simulink model "W06_5_offline"  (R2024b)
settings: Solver=ode4  StartTime=0.0  StopTime=80  FixedStep=0.05  RelTol=1e-3
settings Model: Creator=admin  LastModifiedBy=admin

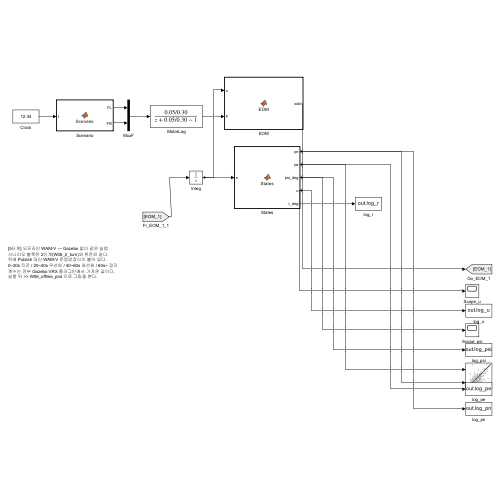
[thumbnail: Simulink's stored preview of the top-level diagram]
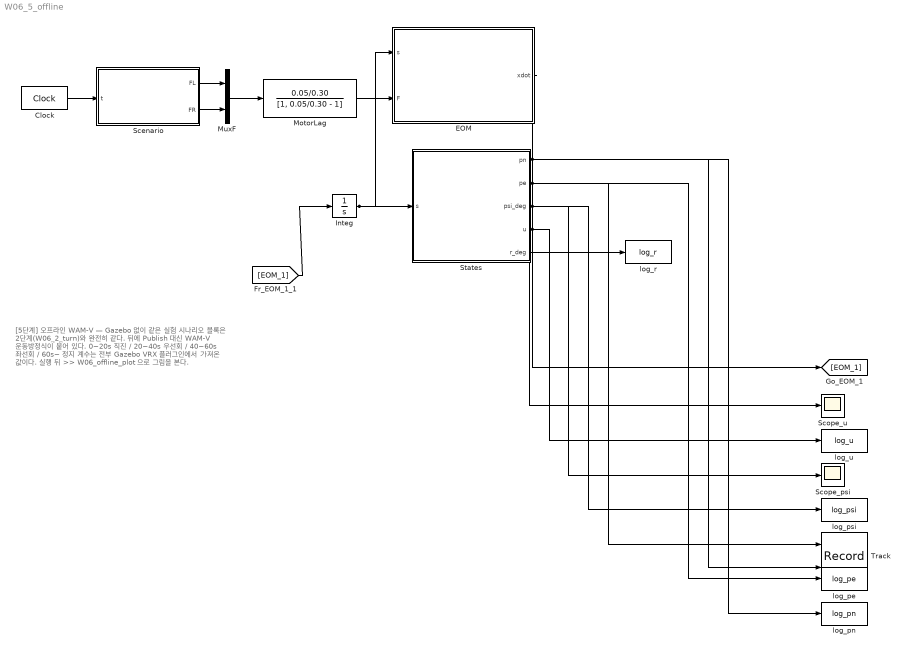
== system W06_5_offline ==
  note: [5단계] 오프라인 WAM-V — Gazebo 없이 같은 실험
      | 시나리오 블록은 2단계(W06_2_turn)와 완전히 같다.
      | 뒤에 Publish 대신 WAM-V 운동방정식이 붙어 있다.
      | 0~20s 직진 / 20~40s 우선회 / 40~60s 좌선회 / 60s~ 정지
      | 계수는 전부 Gazebo VRX 플러그인에서 가져온 값이다.
      | 실행 뒤 >> W06_offline_plot 으로 그림을 본다.
  Clock : DigitalClock  SampleTime=0.05
  EOM : MATLAB Function  TreatAsAtomicUnit=on
  Integ : Integrator  InitialCondition=[0;0;0;0;0;0]
  MotorLag : DiscreteTransferFcn  Numerator=0.05/0.30  Denominator=[1, 0.05/0.30 - 1]  SampleTime=0.05
  MuxF : Mux  Inputs=2
  Scenario : MATLAB Function  TreatAsAtomicUnit=on
  Scope_psi : Scope
  Scope_u : Scope
  States : MATLAB Function  TreatAsAtomicUnit=on
  Track : Record  FileSettingsInternal="{\"entries\":[{\"content\":{\"excelSettings\":{\"content\":{},\"type\":\"Streamout.ExcelSettings\"}},\"type\":\"Streamout.FileSettingStorage\",\"uuid\":\"\"}],\"packageUris\":[\"http:\\/\\/schema.mathworks.com\\/mf0\\/streamout_blocks\\/R2020a\"],\"version\":\"1.0\"}"  Layout=[1 1]  SignalsInternal="{\"entries\":[{\"content\":{\"signals\":[{\"content\":{\"blockPath\":[],\"dimensions\":[1],\"domain\":\"\",\"lineColor\":\"#a2142f\",\"plots\":[ 1 ],\"port\":1,\"signalID\":1,\"signalName\":\"XY Graph:1\"},\"type\":\"RecordBlkView.Signal\",\"uuid\":\"\"},{\"content\":{\"blockPath\":[],\"dimensions\":[1],\"domain\":\"\",\"lineColor\":\"#139fff\",\"plots\":[ 1 ],\"port\":2,\"signalID\":2,\"signalName\":\"XY Graph:2\"},\"type\":\"RecordBlkView.Signal\",\"uuid\":\"\"}]},\"type\":\"RecordBlkView.InputSignals\",\"uuid\":\"\"}],\"packageUris\":[\"http:\\/\\/schema.mathworks.com\\/mf0\\/streamout_blocks\\/R2020a\"],\"version\":\"1.0\"}"  VisualizationBindings="{\"xyplotplugin\":{\"info\":[{\"series\":[{\"bindingParametersList\":[{\"parameter\":\"X-Axis\",\"signalID\":1,\"signalName\":\"XY Graph:1\"},{\"parameter\":\"Y-Axis\",\"signalID\":2,\"signalName\":\"XY Graph:2\"}],\"seriesID\":0}],\"subplotID\":1}]}}"  CompatibilityTag=XY
  log_pe : ToWorkspace  VariableName=log_pe  SaveFormat=Timeseries  SampleTime=0.05
  log_pn : ToWorkspace  VariableName=log_pn  SaveFormat=Timeseries  SampleTime=0.05
  log_psi : ToWorkspace  VariableName=log_psi  SaveFormat=Timeseries  SampleTime=0.05
  log_r : ToWorkspace  VariableName=log_r  SaveFormat=Timeseries  SampleTime=0.05
  log_u : ToWorkspace  VariableName=log_u  SaveFormat=Timeseries  SampleTime=0.05
  wires:
  Clock/1 -> Scenario/1(t)
  Scenario/1(FL) -> MuxF/1
  MotorLag/1 -> EOM/2(F)
  Scenario/2(FR) -> MuxF/2
  MuxF/1 -> MotorLag/1
  Integ/1 -> EOM/1(s), States/1(s)
  States/5(r_deg) -> log_r/1
  [EOM_1] -> Integ/1
  EOM/1(xdot) -> [EOM_1]
  States/4(u) -> Scope_u/1, log_u/1
  States/3(psi_deg) -> Scope_psi/1, log_psi/1
  States/2(pe) -> Track/1, log_pe/1
  States/1(pn) -> Track/2, log_pn/1

== matlab function W06_5_offline/EOM ==
  data: s input; xdot output; F input
function xdot = EOM(s, F)
%#codegen
% 3-DOF WAM-V equations of motion in NED.
% Every coefficient below is taken from the Gazebo VRX plugins, so
% this model and the simulator answer the same question the same way.
%   drag : wamv_gazebo_dynamics_plugin.xacro (SimpleHydrodynamics)
%   mass : wamv_base.urdf.xacro (180 kg hull + 2x15 kg engines)
%   added mass is zero in VRX (xDotU = yDotV = nDotR = 0)
%   s = [u v r N E psi]    F = [FL; FR]

mm  = 211;    Izz = 653;
Xu  = 100;    Xuu = 150;
Yv  = 100;    Yvv = 100;
Nr  = 800;    Nrr = 800;
b   = 1.027135;          % half beam of the aft thrusters [m]

u = s(1); v = s(2); r = s(3); psi = s(6);

% differential thrust -> surge force and yaw moment
X = F(1) + F(2);
N = (F(1) - F(2))*b;

Dx = (Xu + Xuu*abs(u))*u;
Dy = (Yv + Yvv*abs(v))*v;
Dn = (Nr + Nrr*abs(r))*r;

du = (X - Dx)/mm + v*r;     % rigid-body Coriolis
dv = (  - Dy)/mm - u*r;
dr = (N - Dn)/Izz;

xdot = [du; dv; dr;
        u*cos(psi) - v*sin(psi);
        u*sin(psi) + v*cos(psi);
        r];

== matlab function W06_5_offline/Scenario ==
  data: t input; FL output; FR output
function [FL, FR] = Scenario(t)
%#codegen
% Time-based thrust scenario [N] - identical to W06_2_turn
if t < 20
    FL = 200;  FR = 200;   % go straight
elseif t < 40
    FL = 300;  FR =  50;   % turn starboard (right)
elseif t < 60
    FL =  50;  FR = 300;   % turn port (left)
else
    FL = 0;    FR = 0;     % stop
end

== matlab function W06_5_offline/States ==
  data: s input; pn output; pe output; psi_deg output; u output; r_deg output
function [pn, pe, psi_deg, u, r_deg] = States(s)
%#codegen
% Pull the numbers we want to look at out of the state.
pn = s(4);
pe = s(5);
psi_deg = s(6)*180/pi;
u  = s(1);
r_deg = s(3)*180/pi;
